simulink model "velo_id_tc_sl"  (Simulink 7.9)
settings: Solver=FixedStepDiscrete  StartTime=0.0  StopTime=20.0  RelTol=1e-3
values from neighbouring files (symbols this model uses):
  p_const = 0.5    [velo_id_tc.m]
  r_const = 1.3    [velo_id_tc.m]
  ts = 1/50    (= 0.02)    [velo_id_gain.m]    (also in velo_id_tc.m; velo_pi_mbd.m)
  u_ini = 1.5    [velo_id_gain.m]    (also in velo_id_tc.m)
libraries: arduino_io_lib x4
settings Model: Creator=hirata  LastModifiedBy=hirata

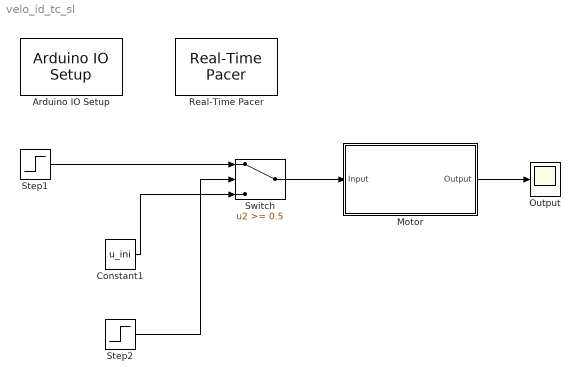
== system velo_id_tc_sl ==
  Arduino IO Setup : arduino_io_lib/Arduino IO Setup  Priority=3  arduinoVar=Arduino1  comPort=COM3
  Constant1 : Constant  Value=u_ini
  Motor : Subsystem
  Output : Scope
      settings: TimeRange=20  YMin=0  YMax=2  SaveName=yout
  Real-Time Pacer : arduino_io_lib/Real-Time Pacer  simTimePerRealTime=1
  Step1 : Step  Time=10  Before=r_const  After=r_const+p_const  SampleTime=ts
  Step2 : Step  SampleTime=ts
  Switch : Switch  Threshold=0.5  SampleTime=ts
  wires:
  Motor/1(Output) -> Output/1
  Constant1/1 -> Switch/3
  Step2/1 -> Switch/2
  Switch/1 -> Motor/1(Input)
  Step1/1 -> Switch/1

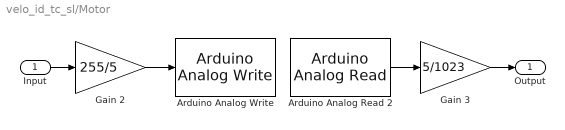
== system velo_id_tc_sl/Motor ==
  Input : Inport
  Arduino Analog Read 2 : arduino_io_lib/Arduino Analog Read  arduinoVar=Arduino1  arduinoPin=0  T=ts
  Arduino Analog Write : arduino_io_lib/Arduino Analog Write  arduinoVar=Arduino1  arduinoPin=3  T=ts
  Gain 2 : Gain  Gain=255/5
  Gain 3 : Gain  Gain=5/1023
  Output : Outport
  wires:
  Arduino Analog Read 2/1 -> Gain 3/1
  Gain 2/1 -> Arduino Analog Write/1
  Input/1 -> Gain 2/1
  Gain 3/1 -> Output/1
